simulink model "Boardinggate_Model"  (R2018a)
settings: Solver=VariableStepAuto  StartTime=0.0  StopTime=10.0  RelTol=1e-3
settings Model: Creator=dell  LastModifiedBy=muhsi
settings CodeAppCC: StateflowObjectComments=on

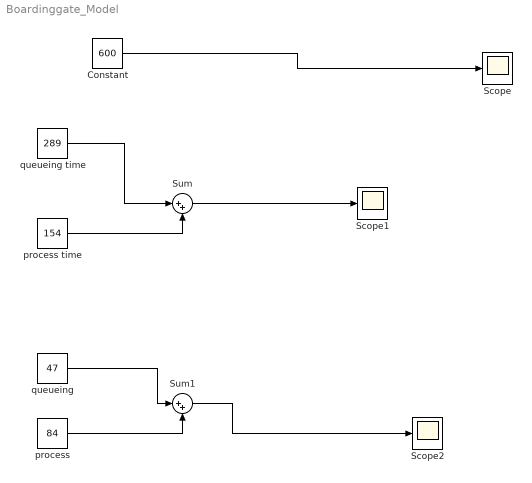
== system Boardinggate_Model ==
  Constant : Constant  Value=600
  Scope : Scope
  Scope1 : Scope
  Scope2 : Scope
  Sum : Sum  Inputs=|++
  Sum1 : Sum  Inputs=|++
  "process " : Constant  Value=84
  "process time " : Constant  Value=154
  "queueing " : Constant  Value=47
  "queueing time " : Constant  Value=289
  wires:
  Constant/1 -> Scope/1
  "process time "/1 -> Sum/2
  "queueing time "/1 -> Sum/1
  Sum1/1 -> Scope2/1
  "process "/1 -> Sum1/2
  "queueing "/1 -> Sum1/1
  Sum/1 -> Scope1/1
